simulink model "SingleStreamSSRwithPL"  (R2021a)
settings: Solver=VariableStepAuto  StartTime=0.0  StopTime=inf  RelTol=1e-3
PreLoadFcn:
  | xmcCheckSlxPath(bdroot)
  | SSR4_init
InitFcn:
  | xmcCheckSlxPath(bdroot)
  | SSR4_init;
undefined symbols (not defined in the file): c, FIR_MultiKernel_cin, FIR_MultiKernel_cincout, FIR_MultiKernel_cout, FramesPerVector, S, SHIFT_ACC, SingleStream, T, Taps, ValidDelay, VectorSize, vsva2197, xcvc1902
libraries: hdlBasic x84, aieBasic x28, simulink x25, aieUtilities x12, dspsrcs4 x1, vmcUtilities x1
(part 3 of 3)

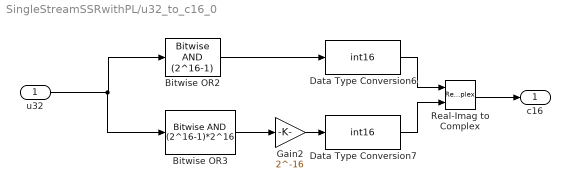
== system SingleStreamSSRwithPL/u32_to_c16_0 ==
  u32 : Inport
  Bitwise OR2 : simulink/Logic and Bit Operations/Bitwise Operator  logicop=AND  UseBitMask=on  BitMask=(2^16-1)  BitMaskRealWorld=Stored Integer
  Bitwise OR3 : simulink/Logic and Bit Operations/Bitwise Operator  logicop=AND  UseBitMask=on  BitMask=(2^16-1)*2^16  BitMaskRealWorld=Stored Integer
  Data Type Conversion6 : DataTypeConversion  OutDataTypeStr=int16  ConvertRealWorld=Stored Integer (SI)
  Data Type Conversion7 : DataTypeConversion  OutDataTypeStr=int16  ConvertRealWorld=Stored Integer (SI)
  Gain2 : Gain  Gain=2^-16  OutDataTypeStr=uint32
  Real-Imag to Complex : RealImagToComplex
  c16 : Outport
  wires:
  u32/1 -> Bitwise OR3/1, Bitwise OR2/1
  Gain2/1 -> Data Type Conversion7/1
  Bitwise OR2/1 -> Data Type Conversion6/1
  Data Type Conversion6/1 -> Real-Imag to Complex/1
  Real-Imag to Complex/1 -> c16/1
  Bitwise OR3/1 -> Gain2/1
  Data Type Conversion7/1 -> Real-Imag to Complex/2

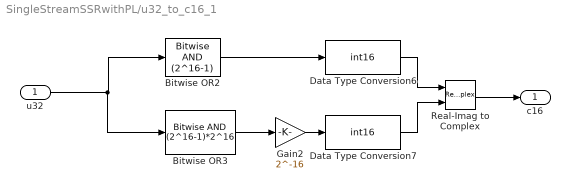
== system SingleStreamSSRwithPL/u32_to_c16_1 ==
  u32 : Inport
  Bitwise OR2 : simulink/Logic and Bit Operations/Bitwise Operator  logicop=AND  UseBitMask=on  BitMask=(2^16-1)  BitMaskRealWorld=Stored Integer
  Bitwise OR3 : simulink/Logic and Bit Operations/Bitwise Operator  logicop=AND  UseBitMask=on  BitMask=(2^16-1)*2^16  BitMaskRealWorld=Stored Integer
  Data Type Conversion6 : DataTypeConversion  OutDataTypeStr=int16  ConvertRealWorld=Stored Integer (SI)
  Data Type Conversion7 : DataTypeConversion  OutDataTypeStr=int16  ConvertRealWorld=Stored Integer (SI)
  Gain2 : Gain  Gain=2^-16  OutDataTypeStr=uint32
  Real-Imag to Complex : RealImagToComplex
  c16 : Outport
  wires:
  Data Type Conversion7/1 -> Real-Imag to Complex/2
  Bitwise OR3/1 -> Gain2/1
  Real-Imag to Complex/1 -> c16/1
  Data Type Conversion6/1 -> Real-Imag to Complex/1
  Bitwise OR2/1 -> Data Type Conversion6/1
  Gain2/1 -> Data Type Conversion7/1
  u32/1 -> Bitwise OR2/1, Bitwise OR3/1

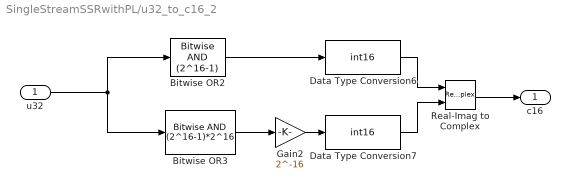
== system SingleStreamSSRwithPL/u32_to_c16_2 ==
  u32 : Inport
  Bitwise OR2 : simulink/Logic and Bit Operations/Bitwise Operator  logicop=AND  UseBitMask=on  BitMask=(2^16-1)  BitMaskRealWorld=Stored Integer
  Bitwise OR3 : simulink/Logic and Bit Operations/Bitwise Operator  logicop=AND  UseBitMask=on  BitMask=(2^16-1)*2^16  BitMaskRealWorld=Stored Integer
  Data Type Conversion6 : DataTypeConversion  OutDataTypeStr=int16  ConvertRealWorld=Stored Integer (SI)
  Data Type Conversion7 : DataTypeConversion  OutDataTypeStr=int16  ConvertRealWorld=Stored Integer (SI)
  Gain2 : Gain  Gain=2^-16  OutDataTypeStr=uint32
  Real-Imag to Complex : RealImagToComplex
  c16 : Outport
  wires:
  u32/1 -> Bitwise OR3/1, Bitwise OR2/1
  Gain2/1 -> Data Type Conversion7/1
  Bitwise OR2/1 -> Data Type Conversion6/1
  Data Type Conversion6/1 -> Real-Imag to Complex/1
  Real-Imag to Complex/1 -> c16/1
  Bitwise OR3/1 -> Gain2/1
  Data Type Conversion7/1 -> Real-Imag to Complex/2

== system SingleStreamSSRwithPL/u32_to_c16_3 ==
  u32 : Inport
  Bitwise OR2 : simulink/Logic and Bit Operations/Bitwise Operator  logicop=AND  UseBitMask=on  BitMask=(2^16-1)  BitMaskRealWorld=Stored Integer
  Bitwise OR3 : simulink/Logic and Bit Operations/Bitwise Operator  logicop=AND  UseBitMask=on  BitMask=(2^16-1)*2^16  BitMaskRealWorld=Stored Integer
  Data Type Conversion6 : DataTypeConversion  OutDataTypeStr=int16  ConvertRealWorld=Stored Integer (SI)
  Data Type Conversion7 : DataTypeConversion  OutDataTypeStr=int16  ConvertRealWorld=Stored Integer (SI)
  Gain2 : Gain  Gain=2^-16  OutDataTypeStr=uint32
  Real-Imag to Complex : RealImagToComplex
  c16 : Outport
  wires:
  Data Type Conversion7/1 -> Real-Imag to Complex/2
  Bitwise OR3/1 -> Gain2/1
  Real-Imag to Complex/1 -> c16/1
  Data Type Conversion6/1 -> Real-Imag to Complex/1
  Bitwise OR2/1 -> Data Type Conversion6/1
  Gain2/1 -> Data Type Conversion7/1
  u32/1 -> Bitwise OR2/1, Bitwise OR3/1

== system SingleStreamSSRwithPL/u32_to_c16_4 ==
  u32 : Inport
  Bitwise OR2 : simulink/Logic and Bit Operations/Bitwise Operator  logicop=AND  UseBitMask=on  BitMask=(2^16-1)  BitMaskRealWorld=Stored Integer
  Bitwise OR3 : simulink/Logic and Bit Operations/Bitwise Operator  logicop=AND  UseBitMask=on  BitMask=(2^16-1)*2^16  BitMaskRealWorld=Stored Integer
  Data Type Conversion6 : DataTypeConversion  OutDataTypeStr=int16  ConvertRealWorld=Stored Integer (SI)
  Data Type Conversion7 : DataTypeConversion  OutDataTypeStr=int16  ConvertRealWorld=Stored Integer (SI)
  Gain2 : Gain  Gain=2^-16  OutDataTypeStr=uint32
  Real-Imag to Complex : RealImagToComplex
  c16 : Outport
  wires:
  u32/1 -> Bitwise OR3/1, Bitwise OR2/1
  Gain2/1 -> Data Type Conversion7/1
  Bitwise OR2/1 -> Data Type Conversion6/1
  Data Type Conversion6/1 -> Real-Imag to Complex/1
  Real-Imag to Complex/1 -> c16/1
  Bitwise OR3/1 -> Gain2/1
  Data Type Conversion7/1 -> Real-Imag to Complex/2

== system SingleStreamSSRwithPL/u32_to_c16_5 ==
  u32 : Inport
  Bitwise OR2 : simulink/Logic and Bit Operations/Bitwise Operator  logicop=AND  UseBitMask=on  BitMask=(2^16-1)  BitMaskRealWorld=Stored Integer
  Bitwise OR3 : simulink/Logic and Bit Operations/Bitwise Operator  logicop=AND  UseBitMask=on  BitMask=(2^16-1)*2^16  BitMaskRealWorld=Stored Integer
  Data Type Conversion6 : DataTypeConversion  OutDataTypeStr=int16  ConvertRealWorld=Stored Integer (SI)
  Data Type Conversion7 : DataTypeConversion  OutDataTypeStr=int16  ConvertRealWorld=Stored Integer (SI)
  Gain2 : Gain  Gain=2^-16  OutDataTypeStr=uint32
  Real-Imag to Complex : RealImagToComplex
  c16 : Outport
  wires:
  Data Type Conversion7/1 -> Real-Imag to Complex/2
  Bitwise OR3/1 -> Gain2/1
  Real-Imag to Complex/1 -> c16/1
  Data Type Conversion6/1 -> Real-Imag to Complex/1
  Bitwise OR2/1 -> Data Type Conversion6/1
  Gain2/1 -> Data Type Conversion7/1
  u32/1 -> Bitwise OR2/1, Bitwise OR3/1

== system SingleStreamSSRwithPL/u32_to_c16_6 ==
  u32 : Inport
  Bitwise OR2 : simulink/Logic and Bit Operations/Bitwise Operator  logicop=AND  UseBitMask=on  BitMask=(2^16-1)  BitMaskRealWorld=Stored Integer
  Bitwise OR3 : simulink/Logic and Bit Operations/Bitwise Operator  logicop=AND  UseBitMask=on  BitMask=(2^16-1)*2^16  BitMaskRealWorld=Stored Integer
  Data Type Conversion6 : DataTypeConversion  OutDataTypeStr=int16  ConvertRealWorld=Stored Integer (SI)
  Data Type Conversion7 : DataTypeConversion  OutDataTypeStr=int16  ConvertRealWorld=Stored Integer (SI)
  Gain2 : Gain  Gain=2^-16  OutDataTypeStr=uint32
  Real-Imag to Complex : RealImagToComplex
  c16 : Outport
  wires:
  u32/1 -> Bitwise OR3/1, Bitwise OR2/1
  Gain2/1 -> Data Type Conversion7/1
  Bitwise OR2/1 -> Data Type Conversion6/1
  Data Type Conversion6/1 -> Real-Imag to Complex/1
  Real-Imag to Complex/1 -> c16/1
  Bitwise OR3/1 -> Gain2/1
  Data Type Conversion7/1 -> Real-Imag to Complex/2

== system SingleStreamSSRwithPL/u32_to_c16_7 ==
  u32 : Inport
  Bitwise OR2 : simulink/Logic and Bit Operations/Bitwise Operator  logicop=AND  UseBitMask=on  BitMask=(2^16-1)  BitMaskRealWorld=Stored Integer
  Bitwise OR3 : simulink/Logic and Bit Operations/Bitwise Operator  logicop=AND  UseBitMask=on  BitMask=(2^16-1)*2^16  BitMaskRealWorld=Stored Integer
  Data Type Conversion6 : DataTypeConversion  OutDataTypeStr=int16  ConvertRealWorld=Stored Integer (SI)
  Data Type Conversion7 : DataTypeConversion  OutDataTypeStr=int16  ConvertRealWorld=Stored Integer (SI)
  Gain2 : Gain  Gain=2^-16  OutDataTypeStr=uint32
  Real-Imag to Complex : RealImagToComplex
  c16 : Outport
  wires:
  Data Type Conversion7/1 -> Real-Imag to Complex/2
  Bitwise OR3/1 -> Gain2/1
  Real-Imag to Complex/1 -> c16/1
  Data Type Conversion6/1 -> Real-Imag to Complex/1
  Bitwise OR2/1 -> Data Type Conversion6/1
  Gain2/1 -> Data Type Conversion7/1
  u32/1 -> Bitwise OR2/1, Bitwise OR3/1

== matlab function SingleStreamSSRwithPL/ComplexSource4/MATLAB Function ==
  data: u input; y1 output; y2 output; y3 output; y4 output; y5 output; y6 output; y7 output; y8 output; valid output; v input
function [y1,y2,y3,y4,y5,y6,y7,y8,valid] = fcn(u,v)


y1 = u(1:8:end);
y2 = u(2:8:end);
y3 = u(3:8:end);
y4 = u(4:8:end);
y5 = u(5:8:end);
y6 = u(6:8:end);
y7 = u(7:8:end);
y8 = u(8:8:end);

valid = v;
